simulink model "fourpost_sim"  (R2020a)
settings: Solver=ode15s  StartTime=0.0  StopTime=T  FixedStep=0.00005  MaxStep=0.0005  RelTol=1e-3  EnableMultiTasking=on
values from neighbouring files (symbols this model uses):
  I_sat = [1/12*m_sat*(3*r^2+h^2),0,0;0,1/12*m_sat*(3*r^2+h^2),0;0,0,1/2*m_sat*r^2]    [berthing_sim_example_run.m]
  kd = 0.00005*[1;1;1;1;1;1;1]    [berthing_sim_example_run.m]
  ki = 0.001*ones(7,1)    [berthing_sim_example_run.m]
  kp = 5*[1;1;1;1;1;1;1]    [berthing_sim_example_run.m]
  m_sat = 2200    [berthing_sim_example_run.m]
  Pd = PBT0    [berthing_sim_example_run.m]
  q0 = [-0.0572;0.8617;0;-1.2870;0.0002;0.4292;0.0570]    [berthing_sim_example_run.m]
  qdot0 = zeros(7,1)    [berthing_sim_example_run.m]
  qlimit = [robot_const(1).limit.lower_joint_limit,     robot_const(1).limit.upper_joint_limit]    [berthing_sim_example_run.m]
  qm0 = robot_const.mprops.N.*q0    [berthing_sim_example_run.m]
  qmdot0 = zeros(7,1)    [berthing_sim_example_run.m]
  r = 0.7    [berthing_sim_example_run.m]
  ts_control = 0.002    [berthing_sim_example_run.m]
undefined symbols (not defined in the file or in its folder): robot_const, rot, X, Y, Z
libraries: sm_lib x63, nesl_utility x43, simulink x7
(part 3 of 3)

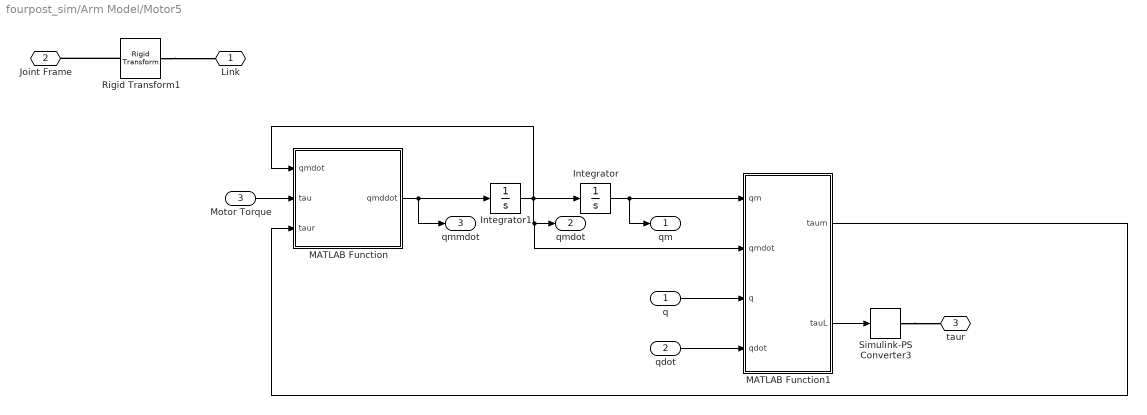
== system fourpost_sim/Arm Model/Motor5 ==
  q : Inport
  qdot : Inport  Port=2
  Motor Torque : Inport  Port=3
  Integrator : Integrator  InitialCondition=qm0
  Integrator1 : Integrator  InitialCondition=qmdot0
  MATLAB Function : MATLAB Function  TreatAsAtomicUnit=on
  MATLAB Function1 : MATLAB Function  TreatAsAtomicUnit=on  mask{N=N, bL=bL, K=K}
      mask prompts: N "Gear Ratio"; bL "Gearbox Friction (Nm s/rad)"; K "Spring Constant (Nm/rad)"
  Rigid Transform1 : sm_lib/Frames and Transforms/Rigid Transform  TranslationMethod=Cartesian  TranslationStandardOffset=0  TranslationLengthUnit=m  TranslationStandardAxis=+Z  TranslationCartesianOffset=rot(h,alpha)*p  TranslationROffset=0  TranslationROffsetUnits=m  TranslationZOffset=0  TranslationZOffsetUnits=m  TranslationThetaOffset=0  TranslationThetaOffsetUnits=deg  RotationMethod=ArbitraryAxis  RotationAngleUnits=rad  RotationStandardAxis=+Z  RotationAngle=alpha  RotationArbitraryAxis=h  FollAlignAxisA=+X  BaseAlignAxisA=+Y  FollAlignAxisB=+Y  BaseAlignAxisB=+Z  RotationSequenceAxes=FollowerAxes  RotationSequence=XYX  RotationSequenceAngles=[0 0 0]  RotationSequenceAnglesUnits=deg  RotationMatrix=[1 0 0; 0 1 0; 0 0 1]
  Simulink-PS Converter3 : nesl_utility/Simulink-PS Converter  PhysicalDomain=network_engine_domain  SubClassName=ps_input  LeftPortType=input  RightPortType=output  PseudoPeriodic=off  Frequencies=[]  NoiseDistribution=none  NoiseParameters=[]  Unit=1  AffineConversion=off  FilteringAndDerivatives=zero  SimscapeFilterOrder=1  InputFilterTimeConstant=0.001  UdotUserProvided=1
  Link : PMIOPort  Side=Right
  Joint Frame : PMIOPort  Port=2  Side=Left
  taur : PMIOPort  Port=3  Side=Right
  qm : Outport  VectorParamsAs1DForOutWhenUnconnected=off
  qmdot : Outport  Port=2  VectorParamsAs1DForOutWhenUnconnected=off
  qmmdot : Outport  Port=3  VectorParamsAs1DForOutWhenUnconnected=off
  wires:
  MATLAB Function1/2(tauL) -> Simulink-PS Converter3/1
  q/1 -> MATLAB Function1/3(q)
  qdot/1 -> MATLAB Function1/4(qdot)
  MATLAB Function1/1(taum) -> MATLAB Function/3(taur)
  Integrator/1 -> qm/1, MATLAB Function1/1(qm)
  Integrator1/1 -> MATLAB Function/1(qmdot), MATLAB Function1/2(qmdot), qmdot/1, Integrator/1
  MATLAB Function/1(qmddot) -> Integrator1/1, qmmdot/1
  Motor Torque/1 -> MATLAB Function/2(tau)
  connections:
  Rigid Transform1/RConn1 -- Link/RConn1
  Rigid Transform1/LConn1 -- Joint Frame/RConn1
  Simulink-PS Converter3/RConn1 -- taur/RConn1

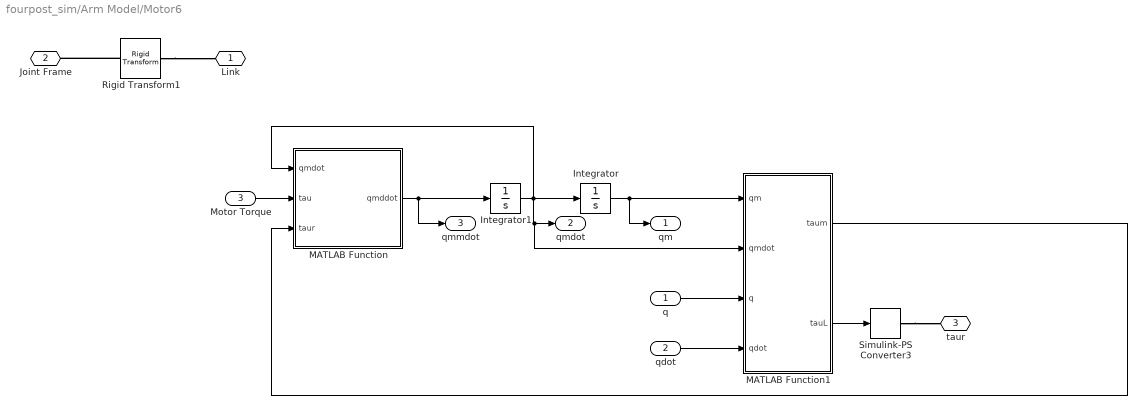
== system fourpost_sim/Arm Model/Motor6 ==
  q : Inport
  qdot : Inport  Port=2
  Motor Torque : Inport  Port=3
  Integrator : Integrator  InitialCondition=qm0
  Integrator1 : Integrator  InitialCondition=qmdot0
  MATLAB Function : MATLAB Function  TreatAsAtomicUnit=on
  MATLAB Function1 : MATLAB Function  TreatAsAtomicUnit=on  mask{N=N, bL=bL, K=K}
      mask prompts: N "Gear Ratio"; bL "Gearbox Friction (Nm s/rad)"; K "Spring Constant (Nm/rad)"
  Rigid Transform1 : sm_lib/Frames and Transforms/Rigid Transform  TranslationMethod=Cartesian  TranslationStandardOffset=0  TranslationLengthUnit=m  TranslationStandardAxis=+Z  TranslationCartesianOffset=p  TranslationROffset=0  TranslationROffsetUnits=m  TranslationZOffset=0  TranslationZOffsetUnits=m  TranslationThetaOffset=0  TranslationThetaOffsetUnits=deg  RotationMethod=ArbitraryAxis  RotationAngleUnits=rad  RotationStandardAxis=+Z  RotationAngle=alpha  RotationArbitraryAxis=h  FollAlignAxisA=+X  BaseAlignAxisA=+Y  FollAlignAxisB=+Y  BaseAlignAxisB=+Z  RotationSequenceAxes=FollowerAxes  RotationSequence=XYX  RotationSequenceAngles=[0 0 0]  RotationSequenceAnglesUnits=deg  RotationMatrix=[1 0 0; 0 1 0; 0 0 1]
  Simulink-PS Converter3 : nesl_utility/Simulink-PS Converter  PhysicalDomain=network_engine_domain  SubClassName=ps_input  LeftPortType=input  RightPortType=output  PseudoPeriodic=off  Frequencies=[]  NoiseDistribution=none  NoiseParameters=[]  Unit=1  AffineConversion=off  FilteringAndDerivatives=zero  SimscapeFilterOrder=1  InputFilterTimeConstant=0.001  UdotUserProvided=1
  Link : PMIOPort  Side=Right
  Joint Frame : PMIOPort  Port=2  Side=Left
  taur : PMIOPort  Port=3  Side=Right
  qm : Outport  VectorParamsAs1DForOutWhenUnconnected=off
  qmdot : Outport  Port=2  VectorParamsAs1DForOutWhenUnconnected=off
  qmmdot : Outport  Port=3  VectorParamsAs1DForOutWhenUnconnected=off
  wires:
  MATLAB Function1/2(tauL) -> Simulink-PS Converter3/1
  q/1 -> MATLAB Function1/3(q)
  qdot/1 -> MATLAB Function1/4(qdot)
  MATLAB Function1/1(taum) -> MATLAB Function/3(taur)
  Integrator/1 -> qm/1, MATLAB Function1/1(qm)
  Integrator1/1 -> MATLAB Function/1(qmdot), MATLAB Function1/2(qmdot), qmdot/1, Integrator/1
  MATLAB Function/1(qmddot) -> Integrator1/1, qmmdot/1
  Motor Torque/1 -> MATLAB Function/2(tau)
  connections:
  Rigid Transform1/RConn1 -- Link/RConn1
  Rigid Transform1/LConn1 -- Joint Frame/RConn1
  Simulink-PS Converter3/RConn1 -- taur/RConn1

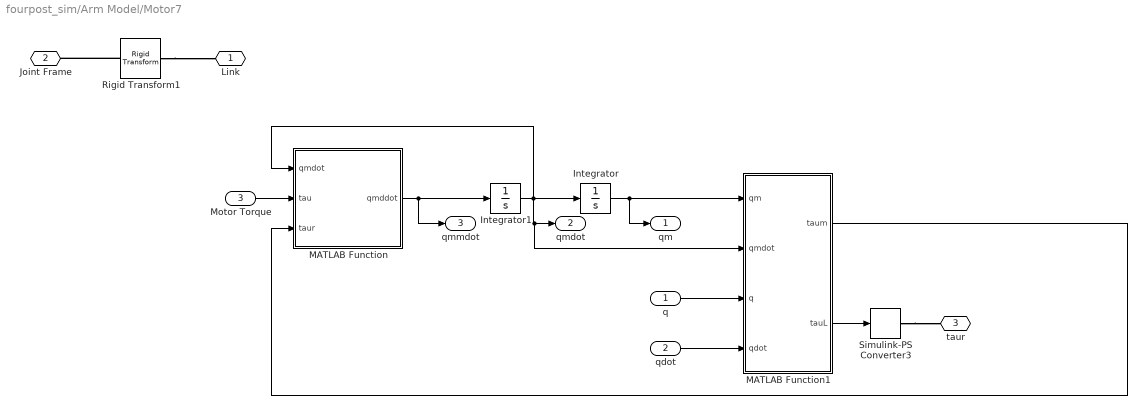
== system fourpost_sim/Arm Model/Motor7 ==
  q : Inport
  qdot : Inport  Port=2
  Motor Torque : Inport  Port=3
  Integrator : Integrator  InitialCondition=qm0
  Integrator1 : Integrator  InitialCondition=qmdot0
  MATLAB Function : MATLAB Function  TreatAsAtomicUnit=on
  MATLAB Function1 : MATLAB Function  TreatAsAtomicUnit=on  mask{N=N, bL=bL, K=K}
      mask prompts: N "Gear Ratio"; bL "Gearbox Friction (Nm s/rad)"; K "Spring Constant (Nm/rad)"
  Rigid Transform1 : sm_lib/Frames and Transforms/Rigid Transform  TranslationMethod=Cartesian  TranslationStandardOffset=0  TranslationLengthUnit=m  TranslationStandardAxis=+Z  TranslationCartesianOffset=rot(h,alpha)*p  TranslationROffset=0  TranslationROffsetUnits=m  TranslationZOffset=0  TranslationZOffsetUnits=m  TranslationThetaOffset=0  TranslationThetaOffsetUnits=deg  RotationMethod=ArbitraryAxis  RotationAngleUnits=rad  RotationStandardAxis=+Z  RotationAngle=alpha  RotationArbitraryAxis=h  FollAlignAxisA=+X  BaseAlignAxisA=+Y  FollAlignAxisB=+Y  BaseAlignAxisB=+Z  RotationSequenceAxes=FollowerAxes  RotationSequence=XYX  RotationSequenceAngles=[0 0 0]  RotationSequenceAnglesUnits=deg  RotationMatrix=[1 0 0; 0 1 0; 0 0 1]
  Simulink-PS Converter3 : nesl_utility/Simulink-PS Converter  PhysicalDomain=network_engine_domain  SubClassName=ps_input  LeftPortType=input  RightPortType=output  PseudoPeriodic=off  Frequencies=[]  NoiseDistribution=none  NoiseParameters=[]  Unit=1  AffineConversion=off  FilteringAndDerivatives=zero  SimscapeFilterOrder=1  InputFilterTimeConstant=0.001  UdotUserProvided=1
  Link : PMIOPort  Side=Right
  Joint Frame : PMIOPort  Port=2  Side=Left
  taur : PMIOPort  Port=3  Side=Right
  qm : Outport  VectorParamsAs1DForOutWhenUnconnected=off
  qmdot : Outport  Port=2  VectorParamsAs1DForOutWhenUnconnected=off
  qmmdot : Outport  Port=3  VectorParamsAs1DForOutWhenUnconnected=off
  wires:
  MATLAB Function1/2(tauL) -> Simulink-PS Converter3/1
  q/1 -> MATLAB Function1/3(q)
  qdot/1 -> MATLAB Function1/4(qdot)
  MATLAB Function1/1(taum) -> MATLAB Function/3(taur)
  Integrator/1 -> qm/1, MATLAB Function1/1(qm)
  Integrator1/1 -> MATLAB Function/1(qmdot), MATLAB Function1/2(qmdot), qmdot/1, Integrator/1
  MATLAB Function/1(qmddot) -> Integrator1/1, qmmdot/1
  Motor Torque/1 -> MATLAB Function/2(tau)
  connections:
  Rigid Transform1/RConn1 -- Link/RConn1
  Rigid Transform1/LConn1 -- Joint Frame/RConn1
  Simulink-PS Converter3/RConn1 -- taur/RConn1

== system fourpost_sim/Controller/C1 ==
  e : Inport
  Discrete PID Controller : simulink/Continuous/PID Controller  Controller=PID  Form=Parallel  TimeDomain=Discrete-time  UseExternalTs=off  SampleTime=ts_control  IntegratorMethod=Forward Euler  FilterMethod=Forward Euler  ControllerParametersSource=internal  P=kp(1)  I=ki(1)  D=kd(1)  UseFilter=on  N=100  TunerSelectOption=Transfer Function Based (PID Tuner App)  InitialConditionSource=internal  InitialConditionForIntegrator=0  InitialConditionForFilter=0  DifferentiatorICPrevScaledInput=0  ExternalReset=none  TrackingMode=off  Kt=1  LimitOutput=off  UpperSaturationLimit=inf  LowerSaturationLimit=-inf  LinearizeAsGain=off  AntiWindupMode=none  Kb=1  POutMin=[]  POutMax=[]  IOutMin=[]  IOutMax=[]  DOutMin=[]  DOutMax=[]  NOutMin=[]  NOutMax=[]  SumOutMin=[]  SumOutMax=[]  SaturationOutMin=[]  SaturationOutMax=[]  PParamMin=[]  PParamMax=[]  IParamMin=[]  IParamMax=[]  DParamMin=[]  DParamMax=[]  NParamMin=[]  NParamMax=[]  KbParamMin=[]  KbParamMax=[]  KtParamMin=[]  KtParamMax=[]  KbOutMin=[]  KbOutMax=[]  KtOutMin=[]  KtOutMax=[]  IntegratorOutMin=[]  IntegratorOutMax=[]  FilterOutMin=[]  FilterOutMax=[]  SumI1OutMin=[]  SumI1OutMax=[]  SumI2OutMin=[]  SumI2OutMax=[]  SumI3OutMin=[]  SumI3OutMax=[]  SumI4OutMin=[]  SumI4OutMax=[]  SumDOutMin=[]  SumDOutMax=[]  DifferentiatorOutMin=[]  DifferentiatorOutMax=[]  FilterDiffOutCoefMin=[]  FilterDiffOutCoefMax=[]  ReciprocalOutMin=[]  ReciprocalOutMax=[]  SumDenOutMin=[]  SumDenOutMax=[]  SumNumOutMin=[]  SumNumOutMax=[]  DivideOutMin=[]  DivideOutMax=[]  UdiffTsProdOutMin=[]  UdiffTsProdOutMax=[]  NTsProdOutMin=[]  NTsProdOutMax=[]  UintegralTsProdOutMin=[]  UintegralTsProdOutMax=[]  UngainTsProdOutMin=[]  UngainTsProdOutMax=[]  IntegratorContinuousStateAttributes=''  IntegratorStateMustResolveToSignalObject=off  IntegratorRTWStateStorageClass=Auto  FilterContinuousStateAttributes=''  FilterStateMustResolveToSignalObject=off  FilterRTWStateStorageClass=Auto  ParallelPVariant=InternalParameters  IdealPVariant=Disabled  IVariant=InternalParameters  DVariant=InternalParameters  IntegratorVariant=Discrete  SatVariant=Disabled  AWVariant=Passthrough  PCopyVariant=Disabled  TRVariant=Disabled  FdbkBlocksVariant=Forward  IdealPFdbkVariant=Disabled  SatFdbkVariant=Disabled  DerivativeFilterVariant=ForwardEulerFilter  NVariant=InternalParameters  NCopyVariant=Disabled  FilterICVariant=InternalICsFilter  IntegratorICVariant=InternalICs  ExternalResetVariant=Disabled  TRSumVariant=Passthrough  SumFdbkVariant=Disabled  SumVariant=Sum_PID  TsampFilterVariant=InternalTs  TsampNgainVariant=Passthrough  TsampIntegralVariant=Passthrough
  Gain : Gain  Gain=robot_const.mprops.N(1)
  tau : Outport  VectorParamsAs1DForOutWhenUnconnected=off
  wires:
  e/1 -> Discrete PID Controller/1
  Gain/1 -> tau/1
  Discrete PID Controller/1 -> Gain/1

== system fourpost_sim/Controller/C2 ==
  e : Inport
  Discrete PID Controller : simulink/Continuous/PID Controller  Controller=PID  Form=Parallel  TimeDomain=Discrete-time  UseExternalTs=off  SampleTime=ts_control  IntegratorMethod=Forward Euler  FilterMethod=Forward Euler  ControllerParametersSource=internal  P=kp(2)  I=ki(2)  D=kd(2)  UseFilter=on  N=100  TunerSelectOption=Transfer Function Based (PID Tuner App)  InitialConditionSource=internal  InitialConditionForIntegrator=0  InitialConditionForFilter=0  DifferentiatorICPrevScaledInput=0  ExternalReset=none  TrackingMode=off  Kt=1  LimitOutput=off  UpperSaturationLimit=inf  LowerSaturationLimit=-inf  LinearizeAsGain=off  AntiWindupMode=none  Kb=1  POutMin=[]  POutMax=[]  IOutMin=[]  IOutMax=[]  DOutMin=[]  DOutMax=[]  NOutMin=[]  NOutMax=[]  SumOutMin=[]  SumOutMax=[]  SaturationOutMin=[]  SaturationOutMax=[]  PParamMin=[]  PParamMax=[]  IParamMin=[]  IParamMax=[]  DParamMin=[]  DParamMax=[]  NParamMin=[]  NParamMax=[]  KbParamMin=[]  KbParamMax=[]  KtParamMin=[]  KtParamMax=[]  KbOutMin=[]  KbOutMax=[]  KtOutMin=[]  KtOutMax=[]  IntegratorOutMin=[]  IntegratorOutMax=[]  FilterOutMin=[]  FilterOutMax=[]  SumI1OutMin=[]  SumI1OutMax=[]  SumI2OutMin=[]  SumI2OutMax=[]  SumI3OutMin=[]  SumI3OutMax=[]  SumI4OutMin=[]  SumI4OutMax=[]  SumDOutMin=[]  SumDOutMax=[]  DifferentiatorOutMin=[]  DifferentiatorOutMax=[]  FilterDiffOutCoefMin=[]  FilterDiffOutCoefMax=[]  ReciprocalOutMin=[]  ReciprocalOutMax=[]  SumDenOutMin=[]  SumDenOutMax=[]  SumNumOutMin=[]  SumNumOutMax=[]  DivideOutMin=[]  DivideOutMax=[]  UdiffTsProdOutMin=[]  UdiffTsProdOutMax=[]  NTsProdOutMin=[]  NTsProdOutMax=[]  UintegralTsProdOutMin=[]  UintegralTsProdOutMax=[]  UngainTsProdOutMin=[]  UngainTsProdOutMax=[]  IntegratorContinuousStateAttributes=''  IntegratorStateMustResolveToSignalObject=off  IntegratorRTWStateStorageClass=Auto  FilterContinuousStateAttributes=''  FilterStateMustResolveToSignalObject=off  FilterRTWStateStorageClass=Auto  ParallelPVariant=InternalParameters  IdealPVariant=Disabled  IVariant=InternalParameters  DVariant=InternalParameters  IntegratorVariant=Discrete  SatVariant=Disabled  AWVariant=Passthrough  PCopyVariant=Disabled  TRVariant=Disabled  FdbkBlocksVariant=Forward  IdealPFdbkVariant=Disabled  SatFdbkVariant=Disabled  DerivativeFilterVariant=ForwardEulerFilter  NVariant=InternalParameters  NCopyVariant=Disabled  FilterICVariant=InternalICsFilter  IntegratorICVariant=InternalICs  ExternalResetVariant=Disabled  TRSumVariant=Passthrough  SumFdbkVariant=Disabled  SumVariant=Sum_PID  TsampFilterVariant=InternalTs  TsampNgainVariant=Passthrough  TsampIntegralVariant=Passthrough
  Gain : Gain  Gain=robot_const.mprops.N(2)
  tau : Outport  VectorParamsAs1DForOutWhenUnconnected=off
  wires:
  e/1 -> Discrete PID Controller/1
  Gain/1 -> tau/1
  Discrete PID Controller/1 -> Gain/1

== system fourpost_sim/Controller/C3 ==
  e : Inport
  Discrete PID Controller : simulink/Continuous/PID Controller  Controller=PID  Form=Parallel  TimeDomain=Discrete-time  UseExternalTs=off  SampleTime=ts_control  IntegratorMethod=Forward Euler  FilterMethod=Forward Euler  ControllerParametersSource=internal  P=kp(3)  I=ki(3)  D=kd(3)  UseFilter=on  N=100  TunerSelectOption=Transfer Function Based (PID Tuner App)  InitialConditionSource=internal  InitialConditionForIntegrator=0  InitialConditionForFilter=0  DifferentiatorICPrevScaledInput=0  ExternalReset=none  TrackingMode=off  Kt=1  LimitOutput=off  UpperSaturationLimit=inf  LowerSaturationLimit=-inf  LinearizeAsGain=off  AntiWindupMode=none  Kb=1  POutMin=[]  POutMax=[]  IOutMin=[]  IOutMax=[]  DOutMin=[]  DOutMax=[]  NOutMin=[]  NOutMax=[]  SumOutMin=[]  SumOutMax=[]  SaturationOutMin=[]  SaturationOutMax=[]  PParamMin=[]  PParamMax=[]  IParamMin=[]  IParamMax=[]  DParamMin=[]  DParamMax=[]  NParamMin=[]  NParamMax=[]  KbParamMin=[]  KbParamMax=[]  KtParamMin=[]  KtParamMax=[]  KbOutMin=[]  KbOutMax=[]  KtOutMin=[]  KtOutMax=[]  IntegratorOutMin=[]  IntegratorOutMax=[]  FilterOutMin=[]  FilterOutMax=[]  SumI1OutMin=[]  SumI1OutMax=[]  SumI2OutMin=[]  SumI2OutMax=[]  SumI3OutMin=[]  SumI3OutMax=[]  SumI4OutMin=[]  SumI4OutMax=[]  SumDOutMin=[]  SumDOutMax=[]  DifferentiatorOutMin=[]  DifferentiatorOutMax=[]  FilterDiffOutCoefMin=[]  FilterDiffOutCoefMax=[]  ReciprocalOutMin=[]  ReciprocalOutMax=[]  SumDenOutMin=[]  SumDenOutMax=[]  SumNumOutMin=[]  SumNumOutMax=[]  DivideOutMin=[]  DivideOutMax=[]  UdiffTsProdOutMin=[]  UdiffTsProdOutMax=[]  NTsProdOutMin=[]  NTsProdOutMax=[]  UintegralTsProdOutMin=[]  UintegralTsProdOutMax=[]  UngainTsProdOutMin=[]  UngainTsProdOutMax=[]  IntegratorContinuousStateAttributes=''  IntegratorStateMustResolveToSignalObject=off  IntegratorRTWStateStorageClass=Auto  FilterContinuousStateAttributes=''  FilterStateMustResolveToSignalObject=off  FilterRTWStateStorageClass=Auto  ParallelPVariant=InternalParameters  IdealPVariant=Disabled  IVariant=InternalParameters  DVariant=InternalParameters  IntegratorVariant=Discrete  SatVariant=Disabled  AWVariant=Passthrough  PCopyVariant=Disabled  TRVariant=Disabled  FdbkBlocksVariant=Forward  IdealPFdbkVariant=Disabled  SatFdbkVariant=Disabled  DerivativeFilterVariant=ForwardEulerFilter  NVariant=InternalParameters  NCopyVariant=Disabled  FilterICVariant=InternalICsFilter  IntegratorICVariant=InternalICs  ExternalResetVariant=Disabled  TRSumVariant=Passthrough  SumFdbkVariant=Disabled  SumVariant=Sum_PID  TsampFilterVariant=InternalTs  TsampNgainVariant=Passthrough  TsampIntegralVariant=Passthrough
  Gain : Gain  Gain=robot_const.mprops.N(3)
  tau : Outport  VectorParamsAs1DForOutWhenUnconnected=off
  wires:
  e/1 -> Discrete PID Controller/1
  Gain/1 -> tau/1
  Discrete PID Controller/1 -> Gain/1

== system fourpost_sim/Controller/C4 ==
  e : Inport
  Discrete PID Controller : simulink/Continuous/PID Controller  Controller=PID  Form=Parallel  TimeDomain=Discrete-time  UseExternalTs=off  SampleTime=ts_control  IntegratorMethod=Forward Euler  FilterMethod=Forward Euler  ControllerParametersSource=internal  P=kp(4)  I=ki(4)  D=kd(4)  UseFilter=on  N=100  TunerSelectOption=Transfer Function Based (PID Tuner App)  InitialConditionSource=internal  InitialConditionForIntegrator=0  InitialConditionForFilter=0  DifferentiatorICPrevScaledInput=0  ExternalReset=none  TrackingMode=off  Kt=1  LimitOutput=off  UpperSaturationLimit=inf  LowerSaturationLimit=-inf  LinearizeAsGain=off  AntiWindupMode=none  Kb=1  POutMin=[]  POutMax=[]  IOutMin=[]  IOutMax=[]  DOutMin=[]  DOutMax=[]  NOutMin=[]  NOutMax=[]  SumOutMin=[]  SumOutMax=[]  SaturationOutMin=[]  SaturationOutMax=[]  PParamMin=[]  PParamMax=[]  IParamMin=[]  IParamMax=[]  DParamMin=[]  DParamMax=[]  NParamMin=[]  NParamMax=[]  KbParamMin=[]  KbParamMax=[]  KtParamMin=[]  KtParamMax=[]  KbOutMin=[]  KbOutMax=[]  KtOutMin=[]  KtOutMax=[]  IntegratorOutMin=[]  IntegratorOutMax=[]  FilterOutMin=[]  FilterOutMax=[]  SumI1OutMin=[]  SumI1OutMax=[]  SumI2OutMin=[]  SumI2OutMax=[]  SumI3OutMin=[]  SumI3OutMax=[]  SumI4OutMin=[]  SumI4OutMax=[]  SumDOutMin=[]  SumDOutMax=[]  DifferentiatorOutMin=[]  DifferentiatorOutMax=[]  FilterDiffOutCoefMin=[]  FilterDiffOutCoefMax=[]  ReciprocalOutMin=[]  ReciprocalOutMax=[]  SumDenOutMin=[]  SumDenOutMax=[]  SumNumOutMin=[]  SumNumOutMax=[]  DivideOutMin=[]  DivideOutMax=[]  UdiffTsProdOutMin=[]  UdiffTsProdOutMax=[]  NTsProdOutMin=[]  NTsProdOutMax=[]  UintegralTsProdOutMin=[]  UintegralTsProdOutMax=[]  UngainTsProdOutMin=[]  UngainTsProdOutMax=[]  IntegratorContinuousStateAttributes=''  IntegratorStateMustResolveToSignalObject=off  IntegratorRTWStateStorageClass=Auto  FilterContinuousStateAttributes=''  FilterStateMustResolveToSignalObject=off  FilterRTWStateStorageClass=Auto  ParallelPVariant=InternalParameters  IdealPVariant=Disabled  IVariant=InternalParameters  DVariant=InternalParameters  IntegratorVariant=Discrete  SatVariant=Disabled  AWVariant=Passthrough  PCopyVariant=Disabled  TRVariant=Disabled  FdbkBlocksVariant=Forward  IdealPFdbkVariant=Disabled  SatFdbkVariant=Disabled  DerivativeFilterVariant=ForwardEulerFilter  NVariant=InternalParameters  NCopyVariant=Disabled  FilterICVariant=InternalICsFilter  IntegratorICVariant=InternalICs  ExternalResetVariant=Disabled  TRSumVariant=Passthrough  SumFdbkVariant=Disabled  SumVariant=Sum_PID  TsampFilterVariant=InternalTs  TsampNgainVariant=Passthrough  TsampIntegralVariant=Passthrough
  Gain : Gain  Gain=robot_const.mprops.N(4)
  tau : Outport  VectorParamsAs1DForOutWhenUnconnected=off
  wires:
  e/1 -> Discrete PID Controller/1
  Gain/1 -> tau/1
  Discrete PID Controller/1 -> Gain/1

== system fourpost_sim/Controller/C5 ==
  e : Inport
  Discrete PID Controller : simulink/Continuous/PID Controller  Controller=PID  Form=Parallel  TimeDomain=Discrete-time  UseExternalTs=off  SampleTime=ts_control  IntegratorMethod=Forward Euler  FilterMethod=Forward Euler  ControllerParametersSource=internal  P=kp(5)  I=ki(5)  D=kd(5)  UseFilter=on  N=100  TunerSelectOption=Transfer Function Based (PID Tuner App)  InitialConditionSource=internal  InitialConditionForIntegrator=0  InitialConditionForFilter=0  DifferentiatorICPrevScaledInput=0  ExternalReset=none  TrackingMode=off  Kt=1  LimitOutput=off  UpperSaturationLimit=inf  LowerSaturationLimit=-inf  LinearizeAsGain=off  AntiWindupMode=none  Kb=1  POutMin=[]  POutMax=[]  IOutMin=[]  IOutMax=[]  DOutMin=[]  DOutMax=[]  NOutMin=[]  NOutMax=[]  SumOutMin=[]  SumOutMax=[]  SaturationOutMin=[]  SaturationOutMax=[]  PParamMin=[]  PParamMax=[]  IParamMin=[]  IParamMax=[]  DParamMin=[]  DParamMax=[]  NParamMin=[]  NParamMax=[]  KbParamMin=[]  KbParamMax=[]  KtParamMin=[]  KtParamMax=[]  KbOutMin=[]  KbOutMax=[]  KtOutMin=[]  KtOutMax=[]  IntegratorOutMin=[]  IntegratorOutMax=[]  FilterOutMin=[]  FilterOutMax=[]  SumI1OutMin=[]  SumI1OutMax=[]  SumI2OutMin=[]  SumI2OutMax=[]  SumI3OutMin=[]  SumI3OutMax=[]  SumI4OutMin=[]  SumI4OutMax=[]  SumDOutMin=[]  SumDOutMax=[]  DifferentiatorOutMin=[]  DifferentiatorOutMax=[]  FilterDiffOutCoefMin=[]  FilterDiffOutCoefMax=[]  ReciprocalOutMin=[]  ReciprocalOutMax=[]  SumDenOutMin=[]  SumDenOutMax=[]  SumNumOutMin=[]  SumNumOutMax=[]  DivideOutMin=[]  DivideOutMax=[]  UdiffTsProdOutMin=[]  UdiffTsProdOutMax=[]  NTsProdOutMin=[]  NTsProdOutMax=[]  UintegralTsProdOutMin=[]  UintegralTsProdOutMax=[]  UngainTsProdOutMin=[]  UngainTsProdOutMax=[]  IntegratorContinuousStateAttributes=''  IntegratorStateMustResolveToSignalObject=off  IntegratorRTWStateStorageClass=Auto  FilterContinuousStateAttributes=''  FilterStateMustResolveToSignalObject=off  FilterRTWStateStorageClass=Auto  ParallelPVariant=InternalParameters  IdealPVariant=Disabled  IVariant=InternalParameters  DVariant=InternalParameters  IntegratorVariant=Discrete  SatVariant=Disabled  AWVariant=Passthrough  PCopyVariant=Disabled  TRVariant=Disabled  FdbkBlocksVariant=Forward  IdealPFdbkVariant=Disabled  SatFdbkVariant=Disabled  DerivativeFilterVariant=ForwardEulerFilter  NVariant=InternalParameters  NCopyVariant=Disabled  FilterICVariant=InternalICsFilter  IntegratorICVariant=InternalICs  ExternalResetVariant=Disabled  TRSumVariant=Passthrough  SumFdbkVariant=Disabled  SumVariant=Sum_PID  TsampFilterVariant=InternalTs  TsampNgainVariant=Passthrough  TsampIntegralVariant=Passthrough
  Gain : Gain  Gain=robot_const.mprops.N(5)
  tau : Outport  VectorParamsAs1DForOutWhenUnconnected=off
  wires:
  e/1 -> Discrete PID Controller/1
  Gain/1 -> tau/1
  Discrete PID Controller/1 -> Gain/1

== system fourpost_sim/Controller/C6 ==
  e : Inport
  Discrete PID Controller : simulink/Continuous/PID Controller  Controller=PID  Form=Parallel  TimeDomain=Discrete-time  UseExternalTs=off  SampleTime=ts_control  IntegratorMethod=Forward Euler  FilterMethod=Forward Euler  ControllerParametersSource=internal  P=kp(6)  I=ki(6)  D=kd(6)  UseFilter=on  N=100  TunerSelectOption=Transfer Function Based (PID Tuner App)  InitialConditionSource=internal  InitialConditionForIntegrator=0  InitialConditionForFilter=0  DifferentiatorICPrevScaledInput=0  ExternalReset=none  TrackingMode=off  Kt=1  LimitOutput=off  UpperSaturationLimit=inf  LowerSaturationLimit=-inf  LinearizeAsGain=off  AntiWindupMode=none  Kb=1  POutMin=[]  POutMax=[]  IOutMin=[]  IOutMax=[]  DOutMin=[]  DOutMax=[]  NOutMin=[]  NOutMax=[]  SumOutMin=[]  SumOutMax=[]  SaturationOutMin=[]  SaturationOutMax=[]  PParamMin=[]  PParamMax=[]  IParamMin=[]  IParamMax=[]  DParamMin=[]  DParamMax=[]  NParamMin=[]  NParamMax=[]  KbParamMin=[]  KbParamMax=[]  KtParamMin=[]  KtParamMax=[]  KbOutMin=[]  KbOutMax=[]  KtOutMin=[]  KtOutMax=[]  IntegratorOutMin=[]  IntegratorOutMax=[]  FilterOutMin=[]  FilterOutMax=[]  SumI1OutMin=[]  SumI1OutMax=[]  SumI2OutMin=[]  SumI2OutMax=[]  SumI3OutMin=[]  SumI3OutMax=[]  SumI4OutMin=[]  SumI4OutMax=[]  SumDOutMin=[]  SumDOutMax=[]  DifferentiatorOutMin=[]  DifferentiatorOutMax=[]  FilterDiffOutCoefMin=[]  FilterDiffOutCoefMax=[]  ReciprocalOutMin=[]  ReciprocalOutMax=[]  SumDenOutMin=[]  SumDenOutMax=[]  SumNumOutMin=[]  SumNumOutMax=[]  DivideOutMin=[]  DivideOutMax=[]  UdiffTsProdOutMin=[]  UdiffTsProdOutMax=[]  NTsProdOutMin=[]  NTsProdOutMax=[]  UintegralTsProdOutMin=[]  UintegralTsProdOutMax=[]  UngainTsProdOutMin=[]  UngainTsProdOutMax=[]  IntegratorContinuousStateAttributes=''  IntegratorStateMustResolveToSignalObject=off  IntegratorRTWStateStorageClass=Auto  FilterContinuousStateAttributes=''  FilterStateMustResolveToSignalObject=off  FilterRTWStateStorageClass=Auto  ParallelPVariant=InternalParameters  IdealPVariant=Disabled  IVariant=InternalParameters  DVariant=InternalParameters  IntegratorVariant=Discrete  SatVariant=Disabled  AWVariant=Passthrough  PCopyVariant=Disabled  TRVariant=Disabled  FdbkBlocksVariant=Forward  IdealPFdbkVariant=Disabled  SatFdbkVariant=Disabled  DerivativeFilterVariant=ForwardEulerFilter  NVariant=InternalParameters  NCopyVariant=Disabled  FilterICVariant=InternalICsFilter  IntegratorICVariant=InternalICs  ExternalResetVariant=Disabled  TRSumVariant=Passthrough  SumFdbkVariant=Disabled  SumVariant=Sum_PID  TsampFilterVariant=InternalTs  TsampNgainVariant=Passthrough  TsampIntegralVariant=Passthrough
  Gain : Gain  Gain=robot_const.mprops.N(6)
  tau : Outport  VectorParamsAs1DForOutWhenUnconnected=off
  wires:
  e/1 -> Discrete PID Controller/1
  Gain/1 -> tau/1
  Discrete PID Controller/1 -> Gain/1

== system fourpost_sim/Controller/C7 ==
  e : Inport
  Discrete PID Controller : simulink/Continuous/PID Controller  Controller=PID  Form=Parallel  TimeDomain=Discrete-time  UseExternalTs=off  SampleTime=ts_control  IntegratorMethod=Forward Euler  FilterMethod=Forward Euler  ControllerParametersSource=internal  P=kp(7)  I=ki(7)  D=kd(7)  UseFilter=on  N=100  TunerSelectOption=Transfer Function Based (PID Tuner App)  InitialConditionSource=internal  InitialConditionForIntegrator=0  InitialConditionForFilter=0  DifferentiatorICPrevScaledInput=0  ExternalReset=none  TrackingMode=off  Kt=1  LimitOutput=off  UpperSaturationLimit=inf  LowerSaturationLimit=-inf  LinearizeAsGain=off  AntiWindupMode=none  Kb=1  POutMin=[]  POutMax=[]  IOutMin=[]  IOutMax=[]  DOutMin=[]  DOutMax=[]  NOutMin=[]  NOutMax=[]  SumOutMin=[]  SumOutMax=[]  SaturationOutMin=[]  SaturationOutMax=[]  PParamMin=[]  PParamMax=[]  IParamMin=[]  IParamMax=[]  DParamMin=[]  DParamMax=[]  NParamMin=[]  NParamMax=[]  KbParamMin=[]  KbParamMax=[]  KtParamMin=[]  KtParamMax=[]  KbOutMin=[]  KbOutMax=[]  KtOutMin=[]  KtOutMax=[]  IntegratorOutMin=[]  IntegratorOutMax=[]  FilterOutMin=[]  FilterOutMax=[]  SumI1OutMin=[]  SumI1OutMax=[]  SumI2OutMin=[]  SumI2OutMax=[]  SumI3OutMin=[]  SumI3OutMax=[]  SumI4OutMin=[]  SumI4OutMax=[]  SumDOutMin=[]  SumDOutMax=[]  DifferentiatorOutMin=[]  DifferentiatorOutMax=[]  FilterDiffOutCoefMin=[]  FilterDiffOutCoefMax=[]  ReciprocalOutMin=[]  ReciprocalOutMax=[]  SumDenOutMin=[]  SumDenOutMax=[]  SumNumOutMin=[]  SumNumOutMax=[]  DivideOutMin=[]  DivideOutMax=[]  UdiffTsProdOutMin=[]  UdiffTsProdOutMax=[]  NTsProdOutMin=[]  NTsProdOutMax=[]  UintegralTsProdOutMin=[]  UintegralTsProdOutMax=[]  UngainTsProdOutMin=[]  UngainTsProdOutMax=[]  IntegratorContinuousStateAttributes=''  IntegratorStateMustResolveToSignalObject=off  IntegratorRTWStateStorageClass=Auto  FilterContinuousStateAttributes=''  FilterStateMustResolveToSignalObject=off  FilterRTWStateStorageClass=Auto  ParallelPVariant=InternalParameters  IdealPVariant=Disabled  IVariant=InternalParameters  DVariant=InternalParameters  IntegratorVariant=Discrete  SatVariant=Disabled  AWVariant=Passthrough  PCopyVariant=Disabled  TRVariant=Disabled  FdbkBlocksVariant=Forward  IdealPFdbkVariant=Disabled  SatFdbkVariant=Disabled  DerivativeFilterVariant=ForwardEulerFilter  NVariant=InternalParameters  NCopyVariant=Disabled  FilterICVariant=InternalICsFilter  IntegratorICVariant=InternalICs  ExternalResetVariant=Disabled  TRSumVariant=Passthrough  SumFdbkVariant=Disabled  SumVariant=Sum_PID  TsampFilterVariant=InternalTs  TsampNgainVariant=Passthrough  TsampIntegralVariant=Passthrough
  Gain : Gain  Gain=robot_const.mprops.N(7)
  tau : Outport  VectorParamsAs1DForOutWhenUnconnected=off
  wires:
  e/1 -> Discrete PID Controller/1
  Gain/1 -> tau/1
  Discrete PID Controller/1 -> Gain/1

== matlab function fourpost_sim/Arm Model/Motor3/MATLAB Function1 ==
  data: qm input; taum output; qmdot input; q input; qdot input; tauL output; K parameter; bL parameter; N parameter
function [taum, tauL] = fnc(qm,qmdot,q,qdot,K, bL, N)

taum = (1/N)*K*(q-(1/N)*qm) + (1/N)*bL*(qdot - (1/N)*qmdot);

tauL = K*((1/N)*qm - q) + bL*((1/N)*qmdot - qdot);

== matlab function fourpost_sim/Arm Model/Motor4/MATLAB Function1 ==
  data: qm input; taum output; qmdot input; q input; qdot input; tauL output; K parameter; bL parameter; N parameter
function [taum, tauL] = fnc(qm,qmdot,q,qdot,K, bL, N)

taum = (1/N)*K*(q-(1/N)*qm) + (1/N)*bL*(qdot - (1/N)*qmdot);

tauL = K*((1/N)*qm - q) + bL*((1/N)*qmdot - qdot);

== matlab function fourpost_sim/Arm Model/Motor5/MATLAB Function ==
  data: qmdot input; qmddot output; tau input; taur input; bm parameter; Jm parameter
function qmddot = fcn(qmdot,tau,taur,bm, Jm)

qmddot = (tau + taur -bm*qmdot)/Jm;

== matlab function fourpost_sim/Arm Model/Motor5/MATLAB Function1 ==
  data: qm input; taum output; qmdot input; q input; qdot input; tauL output; K parameter; bL parameter; N parameter
function [taum, tauL] = fnc(qm,qmdot,q,qdot,K, bL, N)

taum = (1/N)*K*(q-(1/N)*qm) + (1/N)*bL*(qdot - (1/N)*qmdot);

tauL = K*((1/N)*qm - q) + bL*((1/N)*qmdot - qdot);

== matlab function fourpost_sim/Arm Model/Motor6/MATLAB Function1 ==
  data: qm input; taum output; qmdot input; q input; qdot input; tauL output; K parameter; bL parameter; N parameter
function [taum, tauL] = fnc(qm,qmdot,q,qdot,K, bL, N)

taum = (1/N)*K*(q-(1/N)*qm) + (1/N)*bL*(qdot - (1/N)*qmdot);

tauL = K*((1/N)*qm - q) + bL*((1/N)*qmdot - qdot);

== matlab function fourpost_sim/Arm Model/Motor7/MATLAB Function ==
  data: qmdot input; qmddot output; tau input; taur input; bm parameter; Jm parameter
function qmddot = fcn(qmdot,tau,taur,bm, Jm)

qmddot = (tau + taur -bm*qmdot)/Jm;

== matlab function fourpost_sim/Arm Model/Motor3/MATLAB Function ==
  data: qmdot input; qmddot output; tau input; taur input; bm parameter; Jm parameter
function qmddot = fcn(qmdot,tau,taur,bm, Jm)

qmddot = (tau + taur -bm*qmdot)/Jm;

== matlab function fourpost_sim/MATLAB Function ==
  data: q input; qdot output; J input; qlimit input; FEE input; tauEE input; Pd input; P input; R input; r input; VGtaucomp output; debug output
function [qdot,VGtaucomp,debug]  = fcn(q,J,qlimit,FEE,tauEE,Pd,P,R,r)

yawd = 0;
rpy = rotm2eul(R,'XYZ');

fd = 20;
fcomp = FEE(3);
pex = Pd(1)-P(1);
pey = Pd(2)-P(2);
betatau = 1/1500; %1000 %500 almost converges in 100
betaf = 1/1500;


qdot_limit = [-5*ones(7,1),5*ones(7,1)];
lb = [qdot_limit(:,1);0;0]; ub = [qdot_limit(:,2);1;1];

epsilon_r = 0.1;
epsilon_p = 0.1;
c = 0.9;
eta = 0.01;
epsilon_in = 0.15;
e = 0.002;

if (P(3)<1.13)&&(abs(fcomp)>10)
    pg1 = [-0.8*r*sqrt(2);-0.8*r*sqrt(2);0];
    pg2 = [-0.8*r*sqrt(2);0.8*r*sqrt(2);0];
    pg3 = [0.8*r*sqrt(2);0.8*r*sqrt(2);0];
    pg4 = [0.8*r*sqrt(2);-0.8*r*sqrt(2);0];
    pg1_hat = pg1/norm(pg1);
    pg2_hat = pg2/norm(pg2);
    pg3_hat = pg3/norm(pg3);
    pg4_hat = pg4/norm(pg4);
    pg1_hat_perp = [cos(pi/2),-sin(pi/2),0;sin(pi/2),cos(pi/2),0;0 0 1]*pg1_hat;
    pg2_hat_perp = [cos(pi/2),-sin(pi/2),0;sin(pi/2),cos(pi/2),0;0 0 1]*pg2_hat;
    pg3_hat_perp = [cos(pi/2),-sin(pi/2),0;sin(pi/2),cos(pi/2),0;0 0 1]*pg3_hat;
    pg4_hat_perp = [cos(pi/2),-sin(pi/2),0;sin(pi/2),cos(pi/2),0;0 0 1]*pg4_hat;
    taue = zeros(3,1) - [tauEE(1);tauEE(2);0];
    
    
    V1 = [betatau*pg1_hat_perp*dot(taue,pg1_hat_perp);zeros(3,1)];
    AG1 = [R, zeros(3); R*hat(pg1), R];

    V2 = [betatau*pg2_hat_perp*dot(taue,pg2_hat_perp);zeros(3,1)];
    AG2 = [R, zeros(3); R*hat(pg2), R];

    V3 = [betatau*pg3_hat_perp*dot(taue,pg3_hat_perp);zeros(3,1)];
    AG3 = [R, zeros(3); R*hat(pg3), R];

    V4 = [betatau*pg4_hat_perp*dot(taue,pg4_hat_perp);zeros(3,1)];
    AG4 = [R, zeros(3); R*hat(pg4), R];
    
    tau13 = dot(tauEE,[sqrt(2);sqrt(2);0]);
    if tau13>0
        V4 = zeros(6,1);
    elseif tau13<0
        V2 = zeros(6,1);
    end
    
    tau24 = dot(tauEE,[-sqrt(2);sqrt(2);0]);
    if tau24>0
        V3 = zeros(6,1);
    elseif tau24<0
        V1 = zeros(6,1);
    end

    VGtaucomp = AG1*V1 + AG2*V2 + AG3*V3 + AG4*V4;
    debug = 1;
else
    VGtaucomp = zeros(6,1);
    debug = 0;
end


%vr = zeros(3,1);
vr = [0;0;0.1*(yawd-rpy(3))] + VGtaucomp(1:3);
%vt = [0;0;-0.005];
vt = [0.1*pex;0.1*pey;(-fcomp-fd)*betaf] + VGtaucomp(4:6); %4000 % 2000 almost converges in 100

%H = getqp_H(q, J, vr, vt, epsilon_r, epsilon_p);
% Manually compute:
H1 = [J,zeros(6,2)]'*[J,zeros(6,2)];
H2 = [zeros(3,7),vr,zeros(3,1);zeros(3,7),zeros(3,1),vt]'*[zeros(3,7),...
    vr,zeros(3,1);zeros(3,7),zeros(3,1),vt];
H3 = -2*[J,zeros(6,2)]'*[zeros(3,7),vr,zeros(3,1);zeros(3,7),zeros(3,1),vt];
H3 = (H3+H3')/2;
H4 = [zeros(1,7),sqrt(epsilon_r),0;zeros(1,7),0,sqrt(epsilon_p)]'*[zeros(1,7),sqrt(epsilon_r),0;...
    zeros(1,7),0,sqrt(epsilon_p)];
H = 2*(H1+H2+H3+H4);
H = (H+H')/2;

%f = getqp_f( q, epsilon_r, epsilon_p );
f = -2*[zeros(1,7),epsilon_r,epsilon_p]';

h = zeros(14,1);
h(1:7) = q - qlimit(:,1);
h(8:14) = qlimit(:,2) - q;

sigma = inequality_bound(h, c, eta, epsilon_in, e);
dhdq = [eye(7) zeros(7, 2); -eye(7) zeros(7, 2)];

A = -dhdq;
b = -sigma;


opts = optimoptions('quadprog','Algorithm','active-set','Display','off');
[q_prime,~,~] = quadprog(H,f,A,b,[],[],lb,ub,[zeros(7,1);1;1],opts);
qdot = q_prime(1:7);

== matlab function fourpost_sim/Arm Model/Motor7/MATLAB Function1 ==
  data: qm input; taum output; qmdot input; q input; qdot input; tauL output; K parameter; bL parameter; N parameter
function [taum, tauL] = fnc(qm,qmdot,q,qdot,K, bL, N)

taum = (1/N)*K*(q-(1/N)*qm) + (1/N)*bL*(qdot - (1/N)*qmdot);

tauL = K*((1/N)*qm - q) + bL*((1/N)*qmdot - qdot);

== matlab function fourpost_sim/ Forward Kinematics Jacobian/Forward Kinematics Jacobian ==
  data: J output; q input; H parameter; P parameter
function J = robotjacobian(q,H,P)
%#codegen
    n = size(H,2);
    
    p = P(:,1);
    R = eye(3);
    
    hi = zeros(3,n);
    pOi = P;
        
    for i=1:n
        R = R*rot(H(:,i),q(i));
        p = p + R*P(:,i+1);
        pOi(:,i+1) = p;
        hi(:,i) = R*H(:,i);
    end
    
    pOT = pOi(:,end);
    J = zeros(6,n);
    
    for i=1:n
        J(:,i) = [hi(:,i); hat(hi(:,i))*(pOT - pOi(:,i))];
    end
    
end

== matlab function fourpost_sim/Forward Kinematics/Forward Kinematics ==
  data: R output; q input; p output; H parameter; P parameter
function [R, p] = FwdKin(q,H,P)
%#codegen
    n = size(H,2);
    
    p = P(:,1);
    R = eye(3);
        
    for i=1:n
        R = R*rot(H(:,i),q(i));
        p = p + R*P(:,i+1);
    end
    
end

== matlab function fourpost_sim/MATLAB Function1 ==
  data: R input; fEE input; fEEw output; tauEE input; tauEEw output
function [fEEw,tauEEw]  = fcn(R,fEE,tauEE)

% Convert force readings from EE frame to base frame

fEEw = R*fEE;
tauEEw = R*tauEE;

== matlab function fourpost_sim/Arm Model/Motor1/MATLAB Function1 ==
  data: qm input; taum output; qmdot input; q input; qdot input; tauL output; K parameter; bL parameter; N parameter
function [taum, tauL] = fnc(qm,qmdot,q,qdot,K, bL, N)

taum = (1/N)*K*(q-(1/N)*qm) + (1/N)*bL*(qdot - (1/N)*qmdot);

tauL = K*((1/N)*qm - q) + bL*((1/N)*qmdot - qdot);

== matlab function fourpost_sim/Arm Model/Motor4/MATLAB Function ==
  data: qmdot input; qmddot output; tau input; taur input; bm parameter; Jm parameter
function qmddot = fcn(qmdot,tau,taur,bm, Jm)

qmddot = (tau + taur -bm*qmdot)/Jm;

== matlab function fourpost_sim/Arm Model/Motor1/MATLAB Function ==
  data: qmdot input; qmddot output; tau input; taur input; bm parameter; Jm parameter; debug1 output; debug2 output
function [qmddot,debug1,debug2] = fcn(qmdot,tau,taur,bm, Jm)

qmddot = (tau + taur -bm*qmdot)/Jm;

%debug = (taur -bm*qmdot)/Jm;
debug1 = (taur);
%debug = (-bm*qmdot)/Jm;
debug2 = -bm*qmdot;

== matlab function fourpost_sim/Arm Model/Motor6/MATLAB Function ==
  data: qmdot input; qmddot output; tau input; taur input; bm parameter; Jm parameter
function qmddot = fcn(qmdot,tau,taur,bm, Jm)

qmddot = (tau + taur -bm*qmdot)/Jm;

== matlab function fourpost_sim/Arm Model/Motor2/MATLAB Function ==
  data: qmdot input; qmddot output; tau input; taur input; bm parameter; Jm parameter
function qmddot = fcn(qmdot,tau,taur,bm, Jm)

qmddot = (tau + taur -bm*qmdot)/Jm;

== matlab function fourpost_sim/Arm Model/Motor2/MATLAB Function1 ==
  data: qm input; taum output; qmdot input; q input; qdot input; tauL output; K parameter; bL parameter; N parameter
function [taum, tauL] = fnc(qm,qmdot,q,qdot,K, bL, N)

taum = (1/N)*K*(q-(1/N)*qm) + (1/N)*bL*(qdot - (1/N)*qmdot);

tauL = K*((1/N)*qm - q) + bL*((1/N)*qmdot - qdot);
